simulink library "Library_ASK"  (R2018b)
settings: Solver=VariableStepAuto  StartTime=0.0  StopTime=10.0  RelTol=1e-3  EnableMultiTasking=on
undefined symbols (not defined in the file): akt_2GTR_az_HA, akt_2GTR_az_VA, akt_2GTR_rn_HA, akt_2GTR_rn_VA, akt_GTR_az_HA, akt_GTR_az_VA, akt_GTR_rn_HA, akt_GTR_rn_VA, alpha, b_zahn, beta_b, breakpointset, choose_ulg, DiscIntNeverNeededParam, eps_1, eps_2, eps_alpha, eta_aa, eta_Kegel_max, Fx_LSD_max, Fx_mUELG_max, i_DF, i_Kegelrad_OD, i_TRM_G1_HA, i_TRM_G1_VA, i_TRM_G2_HA, i_TRM_G2_VA, i_TRM_HA, i_TRM_Stufe_1_HA, i_TRM_Stufe_1_VA, i_TRM_Stufe_2_HA, i_TRM_Stufe_2_VA, i_TRM_VA, M_Cl_LSD_max, M_Cl_mUELG_max, M_EM_max, M_Kupplung_mUELG_Schlepp, mu_cl_LSD, mu_cl_mUELG, n_EM_max, n_Stufen_TRM_HA, n_Stufen_TRM_VA, ndyn_oil, nreib_LSD, nreib_mUELG, par_MDT, par_VEH, Ra, rm_LSD, rm_mUELG, select_Traktion_split, stepsize, wkg_Diff_mUELG, wkg_GTR, X_L, z_atts, z_ayc, z_ayc_lr, z_ayc_rl
libraries: simulink x23, $bdroot x6
(part 2 of 4)

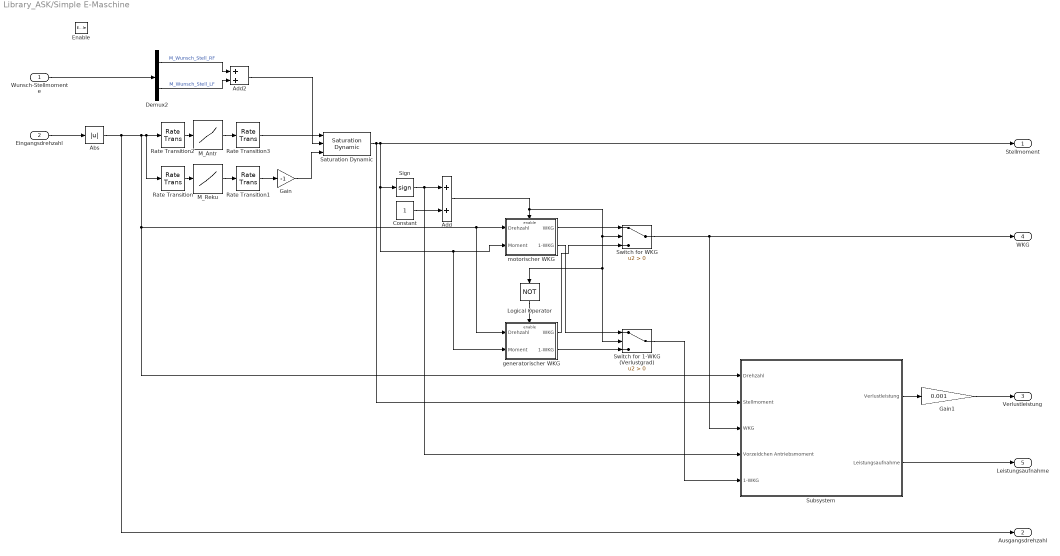
== system Library_ASK/Simple E-Maschine ==
  Wunsch-Stellmomente : Inport
  Eingangsdrehzahl : Inport  Port=2
  Enable : EnablePort
  Abs : Abs
  Add : Sum
  Add2 : Sum
  Constant : Constant
  Demux2 : Demux  Outputs=2
  Gain : Gain  Gain=-1
  Gain1 : Gain  Gain=0.001
  Logical Operator : Logic  Operator=NOT  AllPortsSameDT=off  OutDataTypeStr=boolean
  M_Antr : Lookup_n-D  NumberOfTableDimensions=1  BreakpointsForDimension1=Mot_nmax_Curve  Table=Mot_Mmax_Curve  ExtrapMethod=Clip  UseLastTableValue=on  InternalRulePriority=Speed  RndMeth=Simplest  InputSameDT=on
  M_Reku : Lookup_n-D  NumberOfTableDimensions=1  BreakpointsForDimension1=Gen_nmax_Curve  Table=Gen_Mmax_Curve  ExtrapMethod=Clip  UseLastTableValue=on  InternalRulePriority=Speed  RndMeth=Simplest  InputSameDT=on
  Rate Transition : RateTransition  OutPortSampleTime=stepsize*10
  Rate Transition1 : RateTransition  OutPortSampleTimeOpt=Inherit  OutPortSampleTime=0.001
  Rate Transition2 : RateTransition  OutPortSampleTime=stepsize*10
  Rate Transition3 : RateTransition  OutPortSampleTimeOpt=Inherit  OutPortSampleTime=0.001
  Saturation Dynamic : simulink/Discontinuities/Saturation Dynamic  OutMin=[]  OutMax=[]  OutDataTypeStr=Inherit: Same as second input  OutDataType=fixdt(1, 16)  OutScaling=2^-10  DoSatur=off
  Sign : Signum
  Subsystem : Subsystem
  Switch for 1-WKG (Verlustgrad) : Switch  Criteria=u2 > Threshold
  Switch for WKG : Switch  Criteria=u2 > Threshold
  generatorischer WKG : Subsystem
  motorischer WKG : Subsystem
  Stellmoment : Outport  InitialOutput=0
  Ausgangsdrehzahl : Outport  Port=2  InitialOutput=0
  Verlustleistung : Outport  Port=3
  WKG : Outport  Port=4
  Leistungsaufnahme : Outport  Port=5  InitialOutput=0
  wires:
  Switch for 1-WKG (Verlustgrad)/1 -> Subsystem/5(1-WKG)
  Subsystem/2(Leistungsaufnahme) -> Leistungsaufnahme/1
  Subsystem/1(Verlustleistung) -> Gain1/1
  Switch for WKG/1 -> WKG/1, Subsystem/3(WKG)
  Sign/1 -> Add/1, Subsystem/4(Vorzeidchen Antriebsmoment)
  Abs/1 -> Ausgangsdrehzahl/1, generatorischer WKG/1(Drehzahl), motorischer WKG/1(Drehzahl), Subsystem/1(Drehzahl), Rate Transition2/1, Rate Transition/1
  Logical Operator/1 -> generatorischer WKG/Enable
  Add/1 -> motorischer WKG/Enable, Switch for WKG/2, Logical Operator/1, Switch for 1-WKG (Verlustgrad)/2
  generatorischer WKG/2(1-WKG) -> Switch for 1-WKG (Verlustgrad)/3
  generatorischer WKG/1(WKG) -> Switch for WKG/3
  motorischer WKG/1(WKG) -> Switch for WKG/1
  Constant/1 -> Add/2
  motorischer WKG/2(1-WKG) -> Switch for 1-WKG (Verlustgrad)/1
  Gain/1 -> Saturation Dynamic/3
  Saturation Dynamic/1 -> Stellmoment/1, Sign/1, generatorischer WKG/2(Moment), motorischer WKG/2(Moment), Subsystem/2(Stellmoment)
  Eingangsdrehzahl/1 -> Abs/1
  Add2/1 -> Saturation Dynamic/2
  Demux2/2 -> Add2/2  "M_Wunsch_Stell_LF"
  Demux2/1 -> Add2/1  "M_Wunsch_Stell_RF"
  Wunsch-Stellmomente/1 -> Demux2/1
  Rate Transition3/1 -> Saturation Dynamic/1
  Rate Transition1/1 -> Gain/1
  Rate Transition2/1 -> M_Antr/1
  M_Antr/1 -> Rate Transition3/1
  Rate Transition/1 -> M_Reku/1
  M_Reku/1 -> Rate Transition1/1
  Gain1/1 -> Verlustleistung/1

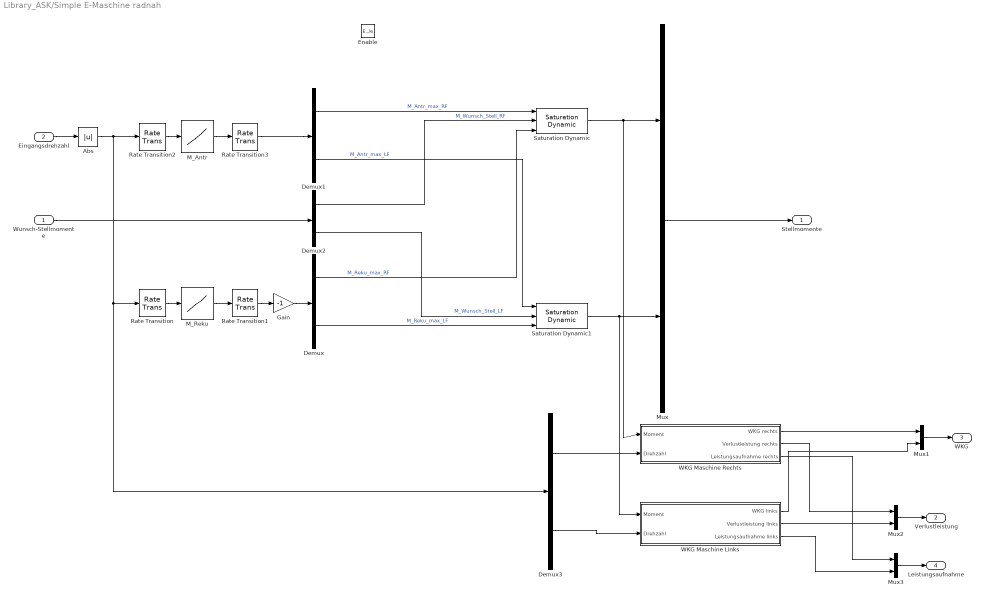
== system Library_ASK/Simple E-Maschine radnah ==
  Wunsch-Stellmomente : Inport
  Eingangsdrehzahl : Inport  Port=2
  Enable : EnablePort
  Abs : Abs
  Demux{,1..3} (4 alike) : Demux  Outputs=2
  Gain : Gain  Gain=-1
  M_Antr : Lookup_n-D  NumberOfTableDimensions=1  BreakpointsForDimension1=Mot_nmax_Curve  Table=Mot_Mmax_Curve  ExtrapMethod=Clip  UseLastTableValue=on  InternalRulePriority=Speed  RndMeth=Simplest  InputSameDT=on
  M_Reku : Lookup_n-D  NumberOfTableDimensions=1  BreakpointsForDimension1=Gen_nmax_Curve  Table=Gen_Mmax_Curve  ExtrapMethod=Clip  UseLastTableValue=on  InternalRulePriority=Speed  RndMeth=Simplest  InputSameDT=on
  Mux{,1..3} (4 alike) : Mux  Inputs=2
  Rate Transition : RateTransition  OutPortSampleTime=stepsize*10
  Rate Transition1 : RateTransition  OutPortSampleTimeOpt=Inherit  OutPortSampleTime=0.001
  Rate Transition2 : RateTransition  OutPortSampleTime=stepsize*10
  Rate Transition3 : RateTransition  OutPortSampleTimeOpt=Inherit  OutPortSampleTime=0.001
  Saturation Dynamic : simulink/Discontinuities/Saturation Dynamic  OutMin=[]  OutMax=[]  OutDataTypeStr=Inherit: Same as second input  OutDataType=fixdt(1, 16)  OutScaling=2^-10  DoSatur=off
  Saturation Dynamic1 : simulink/Discontinuities/Saturation Dynamic  OutMin=[]  OutMax=[]  OutDataTypeStr=Inherit: Same as second input  OutDataType=fixdt(1, 16)  OutScaling=2^-10  DoSatur=off
  WKG Maschine Links : Subsystem
  WKG Maschine Rechts : Subsystem
  Stellmomente : Outport  InitialOutput=0
  Verlustleistung : Outport  Port=2
  WKG : Outport  Port=3
  Leistungsaufnahme : Outport  Port=4
  wires:
  WKG Maschine Links/3(Leistungsaufnahme links) -> Mux3/2
  WKG Maschine Rechts/3(Leistungsaufnahme rechts) -> Mux3/1
  Mux3/1 -> Leistungsaufnahme/1
  Abs/1 -> Rate Transition2/1, Rate Transition/1, Demux3/1
  Mux2/1 -> Verlustleistung/1
  Demux3/2 -> WKG Maschine Links/2(Drehzahl)
  Demux3/1 -> WKG Maschine Rechts/2(Drehzahl)
  Mux1/1 -> WKG/1
  WKG Maschine Links/2(Verlustleistung links) -> Mux2/2
  WKG Maschine Rechts/2(Verlustleistung rechts) -> Mux2/1
  WKG Maschine Rechts/1(WKG rechts) -> Mux1/1
  WKG Maschine Links/1(WKG links) -> Mux1/2
  Gain/1 -> Demux/1
  Eingangsdrehzahl/1 -> Abs/1
  M_Reku/1 -> Rate Transition1/1
  Rate Transition/1 -> M_Reku/1
  M_Antr/1 -> Rate Transition3/1
  Rate Transition2/1 -> M_Antr/1
  Rate Transition1/1 -> Gain/1
  Rate Transition3/1 -> Demux1/1
  Demux/1 -> Saturation Dynamic/3  "M_Reku_max_RF"
  Demux/2 -> Saturation Dynamic1/3  "M_Reku_max_LF"
  Demux1/1 -> Saturation Dynamic/1  "M_Antr_max_RF"
  Demux1/2 -> Saturation Dynamic1/1  "M_Antr_max_LF"
  Wunsch-Stellmomente/1 -> Demux2/1
  Demux2/1 -> Saturation Dynamic/2  "M_Wunsch_Stell_RF"
  Demux2/2 -> Saturation Dynamic1/2  "M_Wunsch_Stell_LF"
  Saturation Dynamic/1 -> Mux/1, WKG Maschine Rechts/1(Moment)
  Saturation Dynamic1/1 -> Mux/2, WKG Maschine Links/1(Moment)
  Mux/1 -> Stellmomente/1

== system Library_ASK/Simple E-Maschine radnah ALT ==
  Wunsch-Stellmomente : Inport
  Eingangsdrehzahl : Inport  Port=2
  Enable : EnablePort
  Abs : Abs
  Demux{,1..3} (4 alike) : Demux  Outputs=2
  Gain : Gain  Gain=-1
  M_Antr : Lookup_n-D  NumberOfTableDimensions=1  BreakpointsForDimension1=Mot_nmax_Curve  Table=Mot_Mmax_Curve  ExtrapMethod=Clip  UseLastTableValue=on  InternalRulePriority=Speed  RndMeth=Simplest  InputSameDT=on
  M_Reku : Lookup_n-D  NumberOfTableDimensions=1  BreakpointsForDimension1=Gen_nmax_Curve  Table=Gen_Mmax_Curve  ExtrapMethod=Clip  UseLastTableValue=on  InternalRulePriority=Speed  RndMeth=Simplest  InputSameDT=on
  Mux{,1..3} (4 alike) : Mux  Inputs=2
  Rate Transition : RateTransition  OutPortSampleTime=stepsize*10
  Rate Transition1 : RateTransition  OutPortSampleTimeOpt=Inherit  OutPortSampleTime=0.001
  Rate Transition2 : RateTransition  OutPortSampleTime=stepsize*10
  Rate Transition3 : RateTransition  OutPortSampleTimeOpt=Inherit  OutPortSampleTime=0.001
  Saturation Dynamic : simulink/Discontinuities/Saturation Dynamic  OutMin=[]  OutMax=[]  OutDataTypeStr=Inherit: Same as second input  OutDataType=fixdt(1, 16)  OutScaling=2^-10  DoSatur=off
  Saturation Dynamic1 : simulink/Discontinuities/Saturation Dynamic  OutMin=[]  OutMax=[]  OutDataTypeStr=Inherit: Same as second input  OutDataType=fixdt(1, 16)  OutScaling=2^-10  DoSatur=off
  WKG Maschine Links : Subsystem
  WKG Maschine Rechts : Subsystem
  Stellmomente : Outport  InitialOutput=0
  Verlustleistung : Outport  Port=2
  WKG : Outport  Port=3
  Leistungsaufnahme : Outport  Port=4
  wires:
  Mux/1 -> Stellmomente/1
  Saturation Dynamic1/1 -> WKG Maschine Links/1(Moment), Mux/2
  Saturation Dynamic/1 -> WKG Maschine Rechts/1(Moment), Mux/1
  Demux2/2 -> Saturation Dynamic1/2  "M_Wunsch_Stell_LF"
  Demux2/1 -> Saturation Dynamic/2  "M_Wunsch_Stell_RF"
  Wunsch-Stellmomente/1 -> Demux2/1
  Demux1/2 -> Saturation Dynamic1/1  "M_Antr_max_LF"
  Demux1/1 -> Saturation Dynamic/1  "M_Antr_max_RF"
  Demux/2 -> Saturation Dynamic1/3  "M_Reku_max_LF"
  Demux/1 -> Saturation Dynamic/3  "M_Reku_max_RF"
  Rate Transition3/1 -> Demux1/1
  Rate Transition1/1 -> Gain/1
  Rate Transition2/1 -> M_Antr/1
  M_Antr/1 -> Rate Transition3/1
  Rate Transition/1 -> M_Reku/1
  M_Reku/1 -> Rate Transition1/1
  Eingangsdrehzahl/1 -> Abs/1
  Gain/1 -> Demux/1
  WKG Maschine Links/1(WKG links) -> Mux1/2
  WKG Maschine Rechts/1(WKG rechts) -> Mux1/1
  WKG Maschine Rechts/2(Verlustleistung rechts) -> Mux2/1
  WKG Maschine Links/2(Verlustleistung links) -> Mux2/2
  Mux1/1 -> WKG/1
  Demux3/1 -> WKG Maschine Rechts/2(Drehzahl)
  Demux3/2 -> WKG Maschine Links/2(Drehzahl)
  Mux2/1 -> Verlustleistung/1
  Abs/1 -> Demux3/1, Rate Transition/1, Rate Transition2/1
  Mux3/1 -> Leistungsaufnahme/1
  WKG Maschine Rechts/3(Leistungsaufnahme rechts) -> Mux3/1
  WKG Maschine Links/3(Leistungsaufnahme links) -> Mux3/2

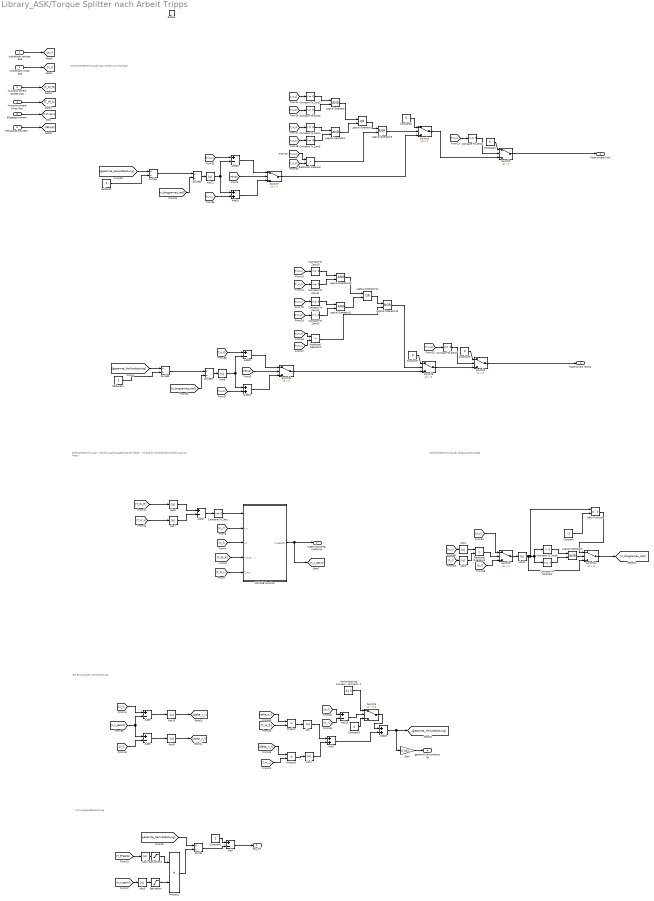
== system Library_ASK/Torque Splitter nach Arbeit Tripps ==
  note: Drehzahlberechnung des langsameren Rades
  note: Drehzahlbestimmung - welche Kupplung geschlossen bleibt - wichtig für die Drehzahlrückführung zum Motor
  note: Berechnung der Verlustleistung
  note: Wirkungsgradberechnung
  note: Momentenberechnung für das rechte und linke Rad
  Istdrehzahl rechtes Rad : Inport
  Istdrehzahl linkes Rad : Inport  Port=2
  Wunschmoment rechtes Rad : Inport  Port=3
  Wunschmoment linkes Rad : Inport  Port=4
  Eingangsmoment : Inport  Port=5
  Rekuperationsindex : Inport  Port=6
  Enable : EnablePort
  Abs{,1..12} (13 alike) : Abs
  Add{,8..9,13,16..17,20} (7 alike) : Sum  Inputs=+-
  Add{7,18..19,21} (4 alike) : Sum
  Compare To Constant : simulink/Logic and Bit Operations/Compare To Constant  relop=<=  const=1  OutDataTypeStr=boolean
  Compare To Zero : simulink/Logic and Bit Operations/Compare To Zero  relop=~=  OutDataTypeStr=boolean
  Compare To Zero1 : simulink/Logic and Bit Operations/Compare To Zero  relop===  OutDataTypeStr=boolean
  Compare To Zero{2..3,10..11} (4 alike) : simulink/Logic and Bit Operations/Compare To Zero  relop=<=  OutDataTypeStr=boolean
  Compare To Zero{4..5,12..13} (4 alike) : simulink/Logic and Bit Operations/Compare To Zero  relop=>=  OutDataTypeStr=boolean
  Compare To Zero7 : simulink/Logic and Bit Operations/Compare To Zero  relop===  OutDataTypeStr=boolean
  Compare To Zero9 : simulink/Logic and Bit Operations/Compare To Zero  relop=>  OutDataTypeStr=boolean
  Constant : Constant  Value=-1
  Constant1 : Constant
  Constant{2,4,6..7,9} (5 alike) : Constant  Value=0
  Divide{,1..3,5} (5 alike) : Product  Inputs=*/
  Gain : Gain  Gain=0.001
  Logical Operator{,1,3,10..11} (5 alike) : Logic  AllPortsSameDT=off  OutDataTypeStr=boolean
  Logical Operator12 : Logic  Operator=OR  AllPortsSameDT=off  OutDataTypeStr=boolean
  Logical Operator13 : Logic  Operator=NOR  AllPortsSameDT=off  OutDataTypeStr=boolean
  Logical Operator2 : Logic  Operator=OR  AllPortsSameDT=off  OutDataTypeStr=boolean
  Logical Operator5 : Logic  Operator=NOR  AllPortsSameDT=off  OutDataTypeStr=boolean
  MATLAB Function : MATLAB Function  TreatAsAtomicUnit=on
  Math Function : Math  Operator=pow  SaturateOnIntegerOverflow=on
  Product : Product
  Product1 : Product
  Product2 : Product
  Relational Operator : RelationalOperator  Operator=>  OutDataTypeStr=boolean  RndMeth=Simplest
  Relational Operator2 : RelationalOperator  Operator=>  OutDataTypeStr=boolean  RndMeth=Simplest
  Relational Operator3 : RelationalOperator  Operator=<  OutDataTypeStr=boolean  RndMeth=Simplest
  Saturation : Saturate  UpperLimit=100000000000  LowerLimit=0.01
  Saturation1 : Saturate  UpperLimit=100000000000  LowerLimit=0.01
  Switch{1..3,6..9,11} (8 alike) : Switch  Criteria=u2 > Threshold
  Switch5 : Switch  Criteria=u2 ~= 0
  "Verlustleistung Aktuierung muss immer aufgebracht werden [W], nur bei Fahrt aktiv 1" : Constant  Value=41.3
  halbieren : Constant  Value=2
  halbieren1 : Constant  Value=2
  Radmoment rechts : Outport
  "Radmoment links " : Outport  Port=2
  n_geschlossene_Kupplung : Outport  Port=3
  gesamte Verlustleistung : Outport  Port=4
  eta_TS : Outport  Port=5
  wires:
  Istdrehzahl linkes Rad/1 -> [n_l]
  Istdrehzahl rechtes Rad/1 -> [n_r]
  Eingangsmoment/1 -> [T_Eingang]
  Wunschmoment rechtes Rad/1 -> [T_W_R]
  Wunschmoment linkes Rad/1 -> [T_W_L]
  [n_l] -> Switch3/3
  [n_r] -> Switch3/1
  Relational Operator3/1 -> Switch3/2
  Switch5/1 -> Add18/1
  [gesamte_Verlustleistung] -> Divide/1
  [delta_n_r] -> Product/1
  [n_k_geschl] -> Add8/1, Add9/2
  [T_Eingang] -> Abs1/1
  [T_W_R] -> Product/2
  [n_l] -> Add8/2
  Abs9/1 -> [delta_n_l]
  "Verlustleistung Aktuierung muss immer aufgebracht werden [W], nur bei Fahrt aktiv 1"/1 -> Switch5/1
  Add/1 -> eta_TS/1
  Product/1 -> Abs/1
  [n_r] -> Add13/2
  [T_W_L] -> Product1/2
  Abs2/1 -> Add7/2
  [n_l] -> Add13/1
  Product1/1 -> Abs2/1
  Abs10/1 -> [delta_n_r]
  [n_r] -> Add9/1
  Constant9/1 -> Switch5/3
  Add18/1 -> Gain/1, [gesamte_Verlustleistung]
  Add7/1 -> Add18/2
  Add9/1 -> Abs10/1
  Constant1/1 -> Add/1
  [delta_n_l] -> Product1/1
  [n_k_geschl] -> Abs3/1
  Product2/1 -> Divide/2
  Add8/1 -> Abs9/1
  Abs/1 -> Add7/1
  Divide/1 -> Add/2
  Add13/1 -> Switch5/2
  [n_langsames_rad] -> Divide3/2
  [T_W_R] -> Add20/1
  [T_W_L] -> Add19/2
  Divide3/1 -> Abs8/1
  Add19/1 -> Switch7/3
  Divide2/1 -> Abs11/1
  halbieren1/1 -> Divide5/2
  [gesamte_Verlustleistung] -> Divide5/1
  Divide5/1 -> Divide3/1
  [T_W_R] -> Add21/2
  Add20/1 -> Switch6/1
  Add16/1 -> Switch7/1
  halbieren/1 -> Divide1/2
  [T_W_L] -> Add16/1
  Add21/1 -> Switch6/3
  [rekup] -> Switch6/2
  [n_langsames_rad] -> Divide2/2
  [rekup] -> Switch7/2
  [gesamte_Verlustleistung] -> Divide1/1
  Divide1/1 -> Divide2/1
  Rekuperationsindex/1 -> [rekup]
  [T_W_L] -> Abs7/1
  Compare To Zero/1 -> MATLAB Function/1(u)
  Add17/1 -> Compare To Zero/1
  MATLAB Function/1(n_k_geschl) -> [n_k_geschl], n_geschlossene_Kupplung/1
  [T_W_R] -> Abs6/1
  Abs6/1 -> Add17/1
  Abs7/1 -> Add17/2
  Gain/1 -> gesamte Verlustleistung/1
  Switch2/1 -> "Radmoment links "/1
  [T_W_R] -> Compare To Zero3/1
  [T_W_R] -> Relational Operator/2
  [T_W_L] -> Compare To Zero2/1
  Logical Operator2/1 -> Logical Operator5/1
  Compare To Zero5/1 -> Logical Operator1/2
  Logical Operator1/1 -> Logical Operator2/2
  [T_W_L] -> Relational Operator/1
  Relational Operator/1 -> Logical Operator5/2
  Compare To Zero3/1 -> Logical Operator/2
  Logical Operator/1 -> Logical Operator2/1
  Constant2/1 -> Switch1/1
  Compare To Zero2/1 -> Logical Operator/1
  [T_W_L] -> Compare To Zero4/1
  Logical Operator5/1 -> Switch1/2
  Switch7/1 -> Switch1/3
  Switch1/1 -> Switch2/3
  Compare To Zero1/1 -> Switch2/2
  [T_W_L] -> Compare To Zero1/1
  [T_W_R] -> Compare To Zero5/1
  Compare To Zero4/1 -> Logical Operator1/1
  Constant4/1 -> Switch2/1
  Switch9/1 -> Radmoment rechts/1
  Compare To Zero7/1 -> Switch9/2
  Constant6/1 -> Switch9/1
  Switch6/1 -> Switch8/3
  Switch8/1 -> Switch9/3
  Logical Operator11/1 -> Logical Operator12/2
  [T_W_L] -> Compare To Zero10/1
  [T_W_R] -> Compare To Zero11/1
  [T_W_R] -> Compare To Zero7/1
  Compare To Zero11/1 -> Logical Operator10/2
  Relational Operator2/1 -> Logical Operator13/2
  Logical Operator12/1 -> Logical Operator13/1
  [T_W_L] -> Compare To Zero12/1
  Logical Operator13/1 -> Switch8/2
  [T_W_R] -> Relational Operator2/1
  Compare To Zero13/1 -> Logical Operator11/2
  Compare To Zero10/1 -> Logical Operator10/1
  Logical Operator10/1 -> Logical Operator12/1
  [T_W_L] -> Relational Operator2/2
  [T_W_R] -> Compare To Zero13/1
  Constant7/1 -> Switch8/1
  Compare To Zero12/1 -> Logical Operator11/1
  Abs3/1 -> Saturation/1
  Saturation/1 -> Product2/2
  Abs1/1 -> Saturation1/1
  Saturation1/1 -> Product2/1
  [n_r] -> Abs4/1
  Abs4/1 -> Relational Operator3/1
  [n_l] -> Abs5/1
  Abs5/1 -> Relational Operator3/2
  [T_W_L] -> MATLAB Function/5(T_W_L)
  [T_W_R] -> MATLAB Function/4(T_W_R)
  [n_l] -> MATLAB Function/3(n_l)
  [n_r] -> MATLAB Function/2(n_r)
  Abs8/1 -> Add21/1, Add20/2
  Abs11/1 -> Add16/2, Add19/1
  Switch3/1 -> Abs12/1
  Compare To Zero9/1 -> Logical Operator3/1
  Compare To Constant/1 -> Logical Operator3/2
  Logical Operator3/1 -> Switch11/2
  Math Function/1 -> Switch11/1
  Constant/1 -> Math Function/2
  Abs12/1 -> Switch11/3, Math Function/1, Compare To Zero9/1, Compare To Constant/1
  Switch11/1 -> [n_langsames_rad]

== system Library_ASK/Torque Splitter v2 C. Angerer 10//2018 ==
  Istdrehzahl rechtes Rad : Inport
  Istdrehzahl linkes Rad : Inport  Port=2
  Wunschmoment rechtes Rad : Inport  Port=3
  Wunschmoment linkes Rad : Inport  Port=4
  Eingangsmoment : Inport  Port=5
  Rekuindex : Inport  Port=6
  Enable : EnablePort
  Constant : Constant  Value=select_Traktion_split
  Gain : Gain  Gain=0.001
  MATLAB Function : MATLAB Function  TreatAsAtomicUnit=on
  MATLAB Function2 : MATLAB Function  TreatAsAtomicUnit=on
  Terminator : Terminator
  Radmoment rechts : Outport
  "Radmoment links " : Outport  Port=2
  n_geschlossene_Kupplung : Outport  Port=3
  gesamte Verlustleistung : Outport  Port=4
  eta_TS : Outport  Port=5
  wires:
  MATLAB Function/3(P_loss_TS) -> Gain/1
  Rekuindex/1 -> Terminator/1
  MATLAB Function/1(M_rad_r) -> Radmoment rechts/1
  MATLAB Function/2(M_rad_l) -> "Radmoment links "/1
  Gain/1 -> gesamte Verlustleistung/1
  MATLAB Function/4(eta_TS) -> eta_TS/1
  MATLAB Function2/1(n_k_geschl) -> n_geschlossene_Kupplung/1, MATLAB Function/6(n_k_geschl)
  Istdrehzahl rechtes Rad/1 -> MATLAB Function2/1(n_r), MATLAB Function/1(n_r)
  Istdrehzahl linkes Rad/1 -> MATLAB Function2/2(n_l), MATLAB Function/2(n_l)
  Wunschmoment rechtes Rad/1 -> MATLAB Function/3(T_W_R)
  Wunschmoment linkes Rad/1 -> MATLAB Function/4(T_W_L)
  Eingangsmoment/1 -> MATLAB Function/5(M_Getriebeausgang), MATLAB Function2/3(Eingangsmoment)
  Constant/1 -> MATLAB Function2/4(split)

== system Library_ASK/Zweigängiges Getriebe az HA ==
  note: Lastanteil
  Eingangsmoment : Inport
  Eingangsdrehzahl : Inport  Port=2
  Enable : EnablePort
  Abs3 : Abs
  Constant : Constant  Value=n_Stufen_TRM_HA
  Constant1 : Constant  Value=M_EM_max
  Constant2 : Constant  Value=i_TRM_G2_HA
  Constant3 : Constant  Value=i_TRM_G1_HA
  Constant5 : Constant  Value=n_EM_max
  Divide : Product  Inputs=*/
  Lastanteil : Product  Inputs=*/
  MATLAB Function : MATLAB Function  TreatAsAtomicUnit=on
  Product : Product  Inputs=3
  Product4 : Product
  Subsystem : Subsystem
  Terminator : Terminator
  WKG : Subsystem
  Ausgangsmoment : Outport  InitialOutput=0
  Energieverlust : Outport  Port=2  InitialOutput=0
  Verlustleistung : Outport  Port=3
  eta_GTR : Outport  Port=4
  wires:
  Constant/1 -> WKG/2(Stufenanzahl)
  MATLAB Function/1(i_TRM) -> WKG/1(Stufenübersetzung), Divide/2, Product/2
  Constant5/1 -> MATLAB Function/2(n_EM_max)
  Constant3/1 -> MATLAB Function/3(i_TRM_G1)
  Constant2/1 -> MATLAB Function/4(i_TRM_G2)
  Eingangsdrehzahl/1 -> MATLAB Function/1(n_EM), Product4/2, Divide/1, WKG/3(Eingangsdrehzahl)
  Subsystem/2(Verlustleistung [kW]) -> Verlustleistung/1
  Subsystem/1(Energieverlust [kWh]) -> Energieverlust/1
  Product4/1 -> Subsystem/2(Inputleistung)  "Electric Motor Input Power [W]"
  Abs3/1 -> WKG/4(Last)
  Constant1/1 -> Lastanteil/2
  Lastanteil/1 -> Abs3/1
  Product/1 -> Ausgangsmoment/1
  Eingangsmoment/1 -> Lastanteil/1, Product/1, Product4/1
  WKG/1(WKG) -> eta_GTR/1, Product/3, Subsystem/1(WKG)
  Divide/1 -> Terminator/1

== system Library_ASK/Zweigängiges Getriebe az VA ==
  note: Lastanteil
  Eingangsmoment : Inport
  Eingangsdrehzahl : Inport  Port=2
  Enable : EnablePort
  Abs3 : Abs
  Constant : Constant  Value=n_Stufen_TRM_VA
  Constant1 : Constant  Value=M_EM_max
  Constant3 : Constant  Value=i_TRM_G1_VA
  Divide : Product  Inputs=*/
  Lastanteil : Product  Inputs=*/
  Product : Product  Inputs=3
  Product4 : Product
  Subsystem : Subsystem
  Terminator : Terminator
  WKG : Subsystem
  Ausgangsmoment : Outport  InitialOutput=0
  Energieverlust : Outport  Port=2  InitialOutput=0
  Verlustleistung : Outport  Port=3
  eta_GTR : Outport  Port=4
  wires:
  Divide/1 -> Terminator/1
  WKG/1(WKG) -> Subsystem/1(WKG), Product/3, eta_GTR/1
  Eingangsmoment/1 -> Product4/1, Product/1, Lastanteil/1
  Product/1 -> Ausgangsmoment/1
  Lastanteil/1 -> Abs3/1
  Constant1/1 -> Lastanteil/2
  Abs3/1 -> WKG/4(Last)
  Product4/1 -> Subsystem/2(Inputleistung)  "Electric Motor Input Power [W]"
  Subsystem/1(Energieverlust [kWh]) -> Energieverlust/1
  Subsystem/2(Verlustleistung [kW]) -> Verlustleistung/1
  Eingangsdrehzahl/1 -> WKG/3(Eingangsdrehzahl), Divide/1, Product4/2
  ? -> ?
  Constant3/1 -> ?
  ? -> Product/2, Divide/2, WKG/1(Stufenübersetzung)
  Constant/1 -> WKG/2(Stufenanzahl)

== system Library_ASK/Zweigängiges Getriebe rn HA ==
  note: Lastanteil
  Eingangsmoment : Inport
  Eingangsdrehzahl : Inport  Port=2
  Enable : EnablePort
  Abs3 : Abs
  Constant : Constant  Value=n_Stufen_TRM_HA
  Constant1 : Constant  Value=M_EM_max
  Constant2 : Constant  Value=i_TRM_G2_HA
  Constant3 : Constant  Value=i_TRM_G1_HA
  Constant5 : Constant  Value=n_EM_max
  Demux : Demux  Outputs=2
  Divide : Product  Inputs=*/
  Lastanteil : Product  Inputs=*/
  MATLAB Function : MATLAB Function  TreatAsAtomicUnit=on
  MATLAB Function1 : MATLAB Function  TreatAsAtomicUnit=on
  Mux : Mux  Inputs=2
  Product : Product  Inputs=3
  Product4 : Product
  Subsystem : Subsystem
  Terminator : Terminator
  WKG : Subsystem
  Ausgangsmoment : Outport  InitialOutput=0
  Energieverlust : Outport  Port=2  InitialOutput=0
  Verlustleistung : Outport  Port=3
  eta_GTR : Outport  Port=4
  wires:
  Mux/1 -> Product/2, Divide/2, WKG/1(Stufenübersetzung)
  MATLAB Function1/1(i_TRM) -> Mux/2
  MATLAB Function/1(i_TRM) -> Mux/1
  Demux/2 -> MATLAB Function1/1(n_EM)
  Demux/1 -> MATLAB Function/1(n_EM)
  Eingangsdrehzahl/1 -> Demux/1, Product4/2, Divide/1, WKG/3(Eingangsdrehzahl)
  Divide/1 -> Terminator/1
  WKG/1(WKG) -> Subsystem/1(WKG), Product/3, eta_GTR/1
  Eingangsmoment/1 -> Lastanteil/1, Product4/1, Product/1
  Product/1 -> Ausgangsmoment/1
  Lastanteil/1 -> Abs3/1
  Constant1/1 -> Lastanteil/2
  Abs3/1 -> WKG/4(Last)
  Product4/1 -> Subsystem/2(Inputleistung)  "Electric Motor Input Power [W]"
  Subsystem/1(Energieverlust [kWh]) -> Energieverlust/1
  Subsystem/2(Verlustleistung [kW]) -> Verlustleistung/1
  Constant2/1 -> MATLAB Function/4(i_TRM_G2), MATLAB Function1/4(i_TRM_G2)
  Constant3/1 -> MATLAB Function/3(i_TRM_G1), MATLAB Function1/3(i_TRM_G1)
  Constant5/1 -> MATLAB Function/2(n_EM_max), MATLAB Function1/2(n_EM_max)
  Constant/1 -> WKG/2(Stufenanzahl)

== system Library_ASK/Zweigängiges Getriebe rn VA ==
  note: Lastanteil
  Eingangsmoment : Inport
  Eingangsdrehzahl : Inport  Port=2
  Enable : EnablePort
  Abs3 : Abs
  Constant : Constant  Value=n_Stufen_TRM_VA
  Constant1 : Constant  Value=M_EM_max
  Constant2 : Constant  Value=i_TRM_G2_VA
  Constant3 : Constant  Value=i_TRM_G1_VA
  Constant5 : Constant  Value=n_EM_max
  Demux : Demux  Outputs=2
  Divide : Product  Inputs=*/
  Lastanteil : Product  Inputs=*/
  MATLAB Function : MATLAB Function  TreatAsAtomicUnit=on
  MATLAB Function1 : MATLAB Function  TreatAsAtomicUnit=on
  Mux : Mux  Inputs=2
  Product : Product  Inputs=3
  Product4 : Product
  Subsystem : Subsystem
  Terminator : Terminator
  WKG : Subsystem
  Ausgangsmoment : Outport  InitialOutput=0
  Energieverlust : Outport  Port=2  InitialOutput=0
  Verlustleistung : Outport  Port=3
  eta_GTR : Outport  Port=4
  wires:
  Constant/1 -> WKG/2(Stufenanzahl)
  Constant5/1 -> MATLAB Function1/2(n_EM_max), MATLAB Function/2(n_EM_max)
  Constant3/1 -> MATLAB Function1/3(i_TRM_G1), MATLAB Function/3(i_TRM_G1)
  Constant2/1 -> MATLAB Function1/4(i_TRM_G2), MATLAB Function/4(i_TRM_G2)
  Subsystem/2(Verlustleistung [kW]) -> Verlustleistung/1
  Subsystem/1(Energieverlust [kWh]) -> Energieverlust/1
  Product4/1 -> Subsystem/2(Inputleistung)  "Electric Motor Input Power [W]"
  Abs3/1 -> WKG/4(Last)
  Constant1/1 -> Lastanteil/2
  Lastanteil/1 -> Abs3/1
  Product/1 -> Ausgangsmoment/1
  Eingangsmoment/1 -> Product/1, Product4/1, Lastanteil/1
  WKG/1(WKG) -> eta_GTR/1, Product/3, Subsystem/1(WKG)
  Divide/1 -> Terminator/1
  Eingangsdrehzahl/1 -> WKG/3(Eingangsdrehzahl), Divide/1, Product4/2, Demux/1
  Demux/1 -> MATLAB Function/1(n_EM)
  Demux/2 -> MATLAB Function1/1(n_EM)
  MATLAB Function/1(i_TRM) -> Mux/1
  MATLAB Function1/1(i_TRM) -> Mux/2
  Mux/1 -> WKG/1(Stufenübersetzung), Divide/2, Product/2

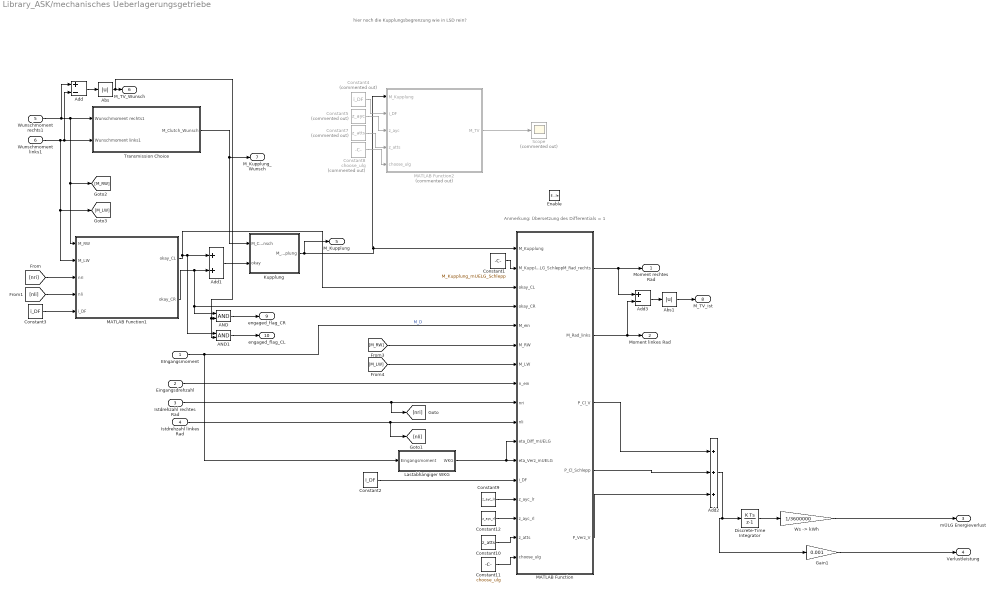
== system Library_ASK/mechanisches Ueberlagerungsgetriebe ==
  note: hier noch die Kupplungsbegrenzung wie in LSD rein?
  note: Anmerkung: Übersetzung des Differentials = 1
  EIngangsmoment : Inport
  Eingangsdrehzahl : Inport  Port=2
  Istdrehzahl rechtes Rad : Inport  Port=3
  Istdrehzahl linkes Rad : Inport  Port=4
  Wunschmoment rechts1 : Inport  Port=5
  Wunschmoment links1 : Inport  Port=6
  Enable : EnablePort
  AND : Logic  IconShape=distinctive  AllPortsSameDT=off  OutDataTypeStr=boolean
  AND1 : Logic  IconShape=distinctive  AllPortsSameDT=off  OutDataTypeStr=boolean
  Abs : Abs
  Abs1 : Abs
  Add : Sum  Inputs=+-
  Add1 : Sum
  Add2 : Sum  Inputs=+++
  Add3 : Sum  Inputs=+-
  Constant1 : Constant  Value=M_Kupplung_mUELG_Schlepp
  Constant10 : Constant  Value=z_atts
  Constant11 : Constant  Value=choose_ulg
  Constant12 : Constant  Value=z_ayc_rl
  Constant2 : Constant  Value=i_DF
  Constant3 : Constant  Value=i_DF
  Constant4 : Constant  Commented=on  Value=i_DF
  Constant5 : Constant  Commented=on  Value=z_ayc
  Constant7 : Constant  Commented=on  Value=z_atts
  Constant8 : Constant  Commented=on  Value=choose_ulg
  Constant9 : Constant  Value=z_ayc_lr
  Discrete-Time Integrator : DiscreteIntegrator  gainval=1  SampleTime=-1  ICPrevOutput=DiscIntNeverNeededParam  ICPrevScaledInput=DiscIntNeverNeededParam
  Gain1 : Gain  Gain=0.001
  Kupplung : Subsystem
  Lastabhängiger WKG : Subsystem
  MATLAB Function : MATLAB Function  TreatAsAtomicUnit=on
  MATLAB Function1 : MATLAB Function  TreatAsAtomicUnit=on
  MATLAB Function2 : MATLAB Function  Commented=on  TreatAsAtomicUnit=on
  Scope : Scope  Commented=on
  Transmission Choice : Subsystem
  "Ws -> kWh" : Gain  Gain=1/3600000
  Moment rechtes Rad : Outport  InitialOutput=0
  Moment linkes Rad : Outport  Port=2  InitialOutput=0
  mÜLG Energieverlust : Outport  Port=3  InitialOutput=0
  Verlustleistung : Outport  Port=4
  M_Kupplung : Outport  Port=5
  M_TV_Wunsch : Outport  Port=6
  M_Kupplung_Wunsch : Outport  Port=7
  M_TV_ist : Outport  Port=8
  engaged_flag_CR : Outport  Port=9
  engaged_flag_CL : Outport  Port=10
  wires:
  MATLAB Function/2(M_Rad_links) -> Add3/2, Moment linkes Rad/1
  MATLAB Function/1(M_Rad_rechts) -> Add3/1, Moment rechtes Rad/1
  Istdrehzahl rechtes Rad/1 -> [nri], MATLAB Function/9(nri)
  Istdrehzahl linkes Rad/1 -> [nli], MATLAB Function/10(nli)
  Constant2/1 -> MATLAB Function/13(i_DF)
  Discrete-Time Integrator/1 -> "Ws -> kWh"/1
  "Ws -> kWh"/1 -> mÜLG Energieverlust/1
  MATLAB Function/3(P_Cl_V) -> Add2/1
  EIngangsmoment/1 -> Lastabhängiger WKG/1(Eingangsmoment), MATLAB Function/5(M_ein)  "M_D"
  Eingangsdrehzahl/1 -> MATLAB Function/8(n_ein)
  Gain1/1 -> Verlustleistung/1
  MATLAB Function1/2(okay_CR) -> Add1/2, AND/1, MATLAB Function/4(okay_CR)
  MATLAB Function1/1(okay_CL) -> MATLAB Function/3(okay_CL), AND1/1, Add1/1
  Add1/1 -> Kupplung/2(okay)
  Kupplung/1(M_Kupplung) -> MATLAB Function2/1(M_Kupplung), MATLAB Function/1(M_Kupplung), M_Kupplung/1
  MATLAB Function/4(P_Cl_Schlepp) -> Add2/2
  MATLAB Function/5(P_Verz_V) -> Add2/3
  Add2/1 -> Gain1/1, Discrete-Time Integrator/1
  [nri] -> MATLAB Function1/3(nri)
  [nli] -> MATLAB Function1/4(nli)
  Constant3/1 -> MATLAB Function1/5(i_DF)
  [M_RW] -> MATLAB Function/6(M_RW)
  [M_LW] -> MATLAB Function/7(M_LW)
  Constant1/1 -> MATLAB Function/2(M_Kupplung_mUELG_Schlepp)
  Wunschmoment rechts1/1 -> Add/1, MATLAB Function1/1(M_RW), [M_RW], Transmission Choice/1(Wunschmoment rechts1)
  Wunschmoment links1/1 -> [M_LW], MATLAB Function1/2(M_LW), Add/2, Transmission Choice/2(Wunschmoment links1)
  Transmission Choice/1(M_Clutch_Wunsch) -> M_Kupplung_Wunsch/1, Kupplung/1(M_Cl_Wunsch)
  Constant4/1 -> MATLAB Function2/2(i_DF)
  Constant5/1 -> MATLAB Function2/3(z_ayc)
  Constant7/1 -> MATLAB Function2/4(z_atts)
  Constant8/1 -> MATLAB Function2/5(choose_ulg)
  Constant9/1 -> MATLAB Function/14(z_ayc_lr)
  Constant10/1 -> MATLAB Function/16(z_atts)
  Constant11/1 -> MATLAB Function/17(choose_ulg)
  MATLAB Function2/1(M_TV) -> Scope/1
  Constant12/1 -> MATLAB Function/15(z_ayc_rl)
  Lastabhängiger WKG/1(WKG) -> MATLAB Function/11(eta_Diff_mUELG), MATLAB Function/12(eta_Verz_mUELG)
  Add/1 -> Abs/1
  Abs/1 -> AND1/2, AND/2, M_TV_Wunsch/1
  Add3/1 -> Abs1/1
  Abs1/1 -> M_TV_ist/1
  AND1/1 -> engaged_flag_CL/1
  AND/1 -> engaged_flag_CR/1

== system Library_ASK/Drehzahlrückführung az HA/Fall Einganggetriebe ==
  Mittlere Raddrehzahl : Inport
  Enable : EnablePort
  Constant : Constant  Value=i_TRM_HA
  Divide : Product  Inputs=**
  Motordrehzahl : Outport
  wires:
  Divide/1 -> Motordrehzahl/1
  Mittlere Raddrehzahl/1 -> Divide/1
  Constant/1 -> Divide/2

== system Library_ASK/Drehzahlrückführung az HA/Fall Zweiganggetriebe ==
  note: auf diese Weise wird die Goto/From - Rückführung aus dem EM -Block überflüssig
  Mittlere Raddrehzahl : Inport
  Enable : EnablePort
  Constant : Constant  Value=i_TRM_G1_HA
  Constant1 : Constant  Value=i_TRM_G2_HA
  Constant2 : Constant  Value=n_EM_max
  Divide : Product  Inputs=**
  Divide1 : Product  Inputs=**
  MATLAB Function : MATLAB Function  TreatAsAtomicUnit=on
  Motordrehzahl : Outport
  wires:
  Constant/1 -> MATLAB Function/3(i_TRM_G1), Divide/2
  Mittlere Raddrehzahl/1 -> Divide/1, Divide1/1
  MATLAB Function/1(i_TRM) -> Divide1/2
  Divide/1 -> MATLAB Function/1(n_EM)  "Motordrehzahl wenn im ersten Gang"
  Constant1/1 -> MATLAB Function/4(i_TRM_G2)
  Divide1/1 -> Motordrehzahl/1
  Constant2/1 -> MATLAB Function/2(n_EM_max)

== system Library_ASK/Drehzahlrückführung az VA/Fall Einganggetriebe ==
  Mittlere Raddrehzahl : Inport
  Enable : EnablePort
  Constant : Constant  Value=i_TRM_VA
  Divide : Product  Inputs=**
  Motordrehzahl : Outport
  wires:
  Constant/1 -> Divide/2
  Mittlere Raddrehzahl/1 -> Divide/1
  Divide/1 -> Motordrehzahl/1

== system Library_ASK/Drehzahlrückführung az VA/Fall Zweiganggetriebe ==
  note: auf diese Weise wird die Goto/From - Rückführung aus dem EM -Block überflüssig
  Mittlere Raddrehzahl : Inport
  Enable : EnablePort
  Constant : Constant  Value=i_TRM_G1_VA
  Constant1 : Constant  Value=i_TRM_G2_VA
  Constant2 : Constant  Value=n_EM_max
  Divide : Product  Inputs=**
  Divide1 : Product  Inputs=**
  MATLAB Function : MATLAB Function  TreatAsAtomicUnit=on
  Motordrehzahl : Outport
  wires:
  Constant2/1 -> MATLAB Function/2(n_EM_max)
  Divide1/1 -> Motordrehzahl/1
  Constant1/1 -> MATLAB Function/4(i_TRM_G2)
  Divide/1 -> MATLAB Function/1(n_EM)  "Motordrehzahl wenn im ersten Gang"
  MATLAB Function/1(i_TRM) -> Divide1/2
  Mittlere Raddrehzahl/1 -> Divide1/1, Divide/1
  Constant/1 -> Divide/2, MATLAB Function/3(i_TRM_G1)

== system Library_ASK/Drehzahlrückführung rn HA/Fall Einganggetriebe ==
  Mittlere Raddrehzahl : Inport
  Enable : EnablePort
  Constant : Constant  Value=i_TRM_HA
  Divide : Product  Inputs=**
  Motordrehzahl : Outport
  wires:
  Constant/1 -> Divide/2
  Mittlere Raddrehzahl/1 -> Divide/1
  Divide/1 -> Motordrehzahl/1

== system Library_ASK/Drehzahlrückführung rn HA/Fall Zweiganggetriebe ==
  note: auf diese Weise wird die Goto/From - Rückführung aus dem EM -Block überflüssig
  note: Das ist jetzt tricky. Denn bei Kurvenfahrt kann es passieren, dass der eine Motor in den zweiten Gang schalten muss, der erste aber nicht.
  Raddrehzahl : Inport
  Enable : EnablePort
  Constant : Constant  Value=i_TRM_G1_HA
  Constant1 : Constant  Value=i_TRM_G2_HA
  Constant2 : Constant  Value=n_EM_max
  Demux : Demux  Outputs=2
  Divide : Product  Inputs=**
  Divide3 : Product  Inputs=**
  MATLAB Function : MATLAB Function  TreatAsAtomicUnit=on
  MATLAB Function1 : MATLAB Function  TreatAsAtomicUnit=on
  Mux : Mux  Inputs=2
  Motordrehzahl : Outport
  wires:
  Mux/1 -> Divide3/2
  Demux/2 -> MATLAB Function1/1(n_EM)  "Motor links"
  Demux/1 -> MATLAB Function/1(n_EM)  "Motor rechts"
  Constant2/1 -> MATLAB Function/2(n_EM_max), MATLAB Function1/2(n_EM_max)
  Constant1/1 -> MATLAB Function/4(i_TRM_G2), MATLAB Function1/4(i_TRM_G2)
  Divide/1 -> Demux/1  "Motordrehzahl wenn im ersten Gang"
  MATLAB Function/1(i_TRM) -> Mux/1
  Raddrehzahl/1 -> Divide3/1, Divide/1
  Constant/1 -> Divide/2, MATLAB Function/3(i_TRM_G1), MATLAB Function1/3(i_TRM_G1)
  MATLAB Function1/1(i_TRM) -> Mux/2
  Divide3/1 -> Motordrehzahl/1

== system Library_ASK/Drehzahlrückführung rn VA/Fall Einganggetriebe ==
  Raddrehzahl : Inport
  Enable : EnablePort
  Constant : Constant  Value=i_TRM_VA
  Divide : Product  Inputs=**
  Motordrehzahl : Outport
  wires:
  Divide/1 -> Motordrehzahl/1
  Raddrehzahl/1 -> Divide/1
  Constant/1 -> Divide/2

== system Library_ASK/Drehzahlrückführung rn VA/Fall Zweiganggetriebe ==
  note: Das ist jetzt tricky. Denn bei Kurvenfahrt kann es passieren, dass der eine Motor in den zweiten Gang schalten muss, der erste aber nicht.
  note: auf diese Weise wird die Goto/From - Rückführung aus dem EM -Block überflüssig
  Raddrehzahl : Inport
  Enable : EnablePort
  Constant : Constant  Value=i_TRM_G1_VA
  Constant1 : Constant  Value=i_TRM_G2_VA
  Constant2 : Constant  Value=n_EM_max
  Demux : Demux  Outputs=2
  Divide : Product  Inputs=**
  Divide2 : Product  Inputs=**
  MATLAB Function : MATLAB Function  TreatAsAtomicUnit=on
  MATLAB Function1 : MATLAB Function  TreatAsAtomicUnit=on
  Mux : Mux  Inputs=2
  Motordrehzahl : Outport
  wires:
  Constant/1 -> MATLAB Function1/3(i_TRM_G1), MATLAB Function/3(i_TRM_G1), Divide/2
  Raddrehzahl/1 -> Divide2/1, Divide/1
  MATLAB Function/1(i_TRM) -> Mux/1
  Divide/1 -> Demux/1  "Motordrehzahl wenn im ersten Gang"
  Constant1/1 -> MATLAB Function1/4(i_TRM_G2), MATLAB Function/4(i_TRM_G2)
  Constant2/1 -> MATLAB Function1/2(n_EM_max), MATLAB Function/2(n_EM_max)
  Demux/1 -> MATLAB Function/1(n_EM)  "Motor rechts"
  Demux/2 -> MATLAB Function1/1(n_EM)  "Motor links"
  Mux/1 -> Divide2/2
  MATLAB Function1/1(i_TRM) -> Mux/2
  Divide2/1 -> Motordrehzahl/1

== system Library_ASK/Elektrisches Überlagerungsgetriebe HA/Momentenkennlinie SEM ==
  Maximalmoment : Inport
  Drehzahl SteuerEM : Inport  Port=2
  Gain : Gain  Gain=-1
  M_Antr : Lookup_n-D  NumberOfTableDimensions=1  BreakpointsForDimension1=par_MDT.HA.trans.etv.Kennfelder.MaxMotorTrqCurve_w  Table=par_MDT.HA.trans.etv.Kennfelder.MaxMotorTrqCurve_M  ExtrapMethod=Clip  UseLastTableValue=on  InternalRulePriority=Speed  RndMeth=Simplest  InputSameDT=on
  M_Reku : Lookup_n-D  NumberOfTableDimensions=1  BreakpointsForDimension1=par_MDT.HA.trans.etv.Kennfelder.MaxGeneratorTrqCurve_w  Table=par_MDT.HA.trans.etv.Kennfelder.MaxGeneratorTrqCurve_M  ExtrapMethod=Clip  UseLastTableValue=on  InternalRulePriority=Speed  RndMeth=Simplest  InputSameDT=on
  Saturation Dynamic : simulink/Discontinuities/Saturation Dynamic  OutMin=[]  OutMax=[]  OutDataTypeStr=Inherit: Same as second input  OutDataType=fixdt(1, 16)  OutScaling=2^-10  DoSatur=off
  Maximalmoment bei Drehzahl : Outport
  wires:
  M_Antr/1 -> Saturation Dynamic/1
  Drehzahl SteuerEM/1 -> M_Antr/1, M_Reku/1
  Gain/1 -> Saturation Dynamic/3
  Maximalmoment/1 -> Saturation Dynamic/2
  Saturation Dynamic/1 -> Maximalmoment bei Drehzahl/1
  M_Reku/1 -> Gain/1

== system Library_ASK/Elektrisches Überlagerungsgetriebe HA/eUELG Steuermaschine ==
  Moment : Inport
  Drehzahl : Inport  Port=2
  Abs : Abs
  Abs1 : Abs
  Wirkungsgradkennfeld nach Pesce : Lookup_n-D  BreakpointsForDimension1=par_MDT.HA.trans.etv.Kennfelder.MotorEffMap3D_w  BreakpointsForDimension2=par_MDT.HA.trans.etv.Kennfelder.MotorEffMap3D_M  Table=par_MDT.HA.trans.etv.Kennfelder.MotorEffMap3D  ExtrapMethod=Clip  UseLastTableValue=on  InternalRulePriority=Speed  RndMeth=Simplest  InputSameDT=on
  Wirkungsgrad : Outport  InitialOutput=0
  wires:
  Moment/1 -> Abs/1
  Drehzahl/1 -> Abs1/1
  Wirkungsgradkennfeld nach Pesce/1 -> Wirkungsgrad/1
  Abs/1 -> Wirkungsgradkennfeld nach Pesce/2
  Abs1/1 -> Wirkungsgradkennfeld nach Pesce/1

== system Library_ASK/Elektrisches Überlagerungsgetriebe VA/Momentenkennlinie SEM ==
  Maximalmoment : Inport
  Drehzahl SteuerEM : Inport  Port=2
  Gain : Gain  Gain=-1
  M_Antr : Lookup_n-D  NumberOfTableDimensions=1  BreakpointsForDimension1=par_MDT.VA.trans.etv.Kennfelder.MaxMotorTrqCurve_w  Table=par_MDT.VA.trans.etv.Kennfelder.MaxMotorTrqCurve_M  ExtrapMethod=Clip  UseLastTableValue=on  InternalRulePriority=Speed  RndMeth=Simplest  InputSameDT=on
  M_Reku : Lookup_n-D  NumberOfTableDimensions=1  BreakpointsForDimension1=par_MDT.VA.trans.etv.Kennfelder.MaxGeneratorTrqCurve_w  Table=par_MDT.VA.trans.etv.Kennfelder.MaxGeneratorTrqCurve_M  ExtrapMethod=Clip  UseLastTableValue=on  InternalRulePriority=Speed  RndMeth=Simplest  InputSameDT=on
  Saturation Dynamic : simulink/Discontinuities/Saturation Dynamic  OutMin=[]  OutMax=[]  OutDataTypeStr=Inherit: Same as second input  OutDataType=fixdt(1, 16)  OutScaling=2^-10  DoSatur=off
  Maximalmoment bei Drehzahl : Outport
  wires:
  M_Reku/1 -> Gain/1
  Saturation Dynamic/1 -> Maximalmoment bei Drehzahl/1
  Maximalmoment/1 -> Saturation Dynamic/2
  Gain/1 -> Saturation Dynamic/3
  Drehzahl SteuerEM/1 -> M_Reku/1, M_Antr/1
  M_Antr/1 -> Saturation Dynamic/1

== system Library_ASK/Elektrisches Überlagerungsgetriebe VA/eUELG Steuermaschine ==
  Moment : Inport
  Drehzahl : Inport  Port=2
  Abs : Abs
  Abs1 : Abs
  Wirkungsgradkennfeld nach Pesce : Lookup_n-D  BreakpointsForDimension1=par_MDT.VA.trans.etv.Kennfelder.MotorEffMap3D_w  BreakpointsForDimension2=par_MDT.VA.trans.etv.Kennfelder.MotorEffMap3D_M  Table=par_MDT.VA.trans.etv.Kennfelder.MotorEffMap3D  ExtrapMethod=Clip  UseLastTableValue=on  InternalRulePriority=Speed  RndMeth=Simplest  InputSameDT=on
  Wirkungsgrad : Outport  InitialOutput=0
  wires:
  Abs1/1 -> Wirkungsgradkennfeld nach Pesce/1
  Abs/1 -> Wirkungsgradkennfeld nach Pesce/2
  Wirkungsgradkennfeld nach Pesce/1 -> Wirkungsgrad/1
  Drehzahl/1 -> Abs1/1
  Moment/1 -> Abs/1

== system Library_ASK/Kelly/x-Achsen-Parameter ==
  note: Umfangskraft Planententeilkreis
  Drehzahl Planet : Inport
  Teilkreis Planet : Inport  Port=2
  Stegmoment : Inport  Port=3
  Durchmesser Steg : Inport  Port=4
  Constant1 : Constant  Value=2
  Divide1 : Product  Inputs=*/
  Eingriffswinkel : Constant  Value=alpha
  Gain2 : Gain  Gain=0.5
  "N/mm -> lb/in" : Gain  Gain=5.71
  "Nm -> Nmm" : Gain  Gain=1000
  Product : Product  Inputs=3
  Product3 : Product
  Summengeschwindigkeit : Product  Inputs=3
  Trigonometric Function1 : Trigonometry
  Zahnbreite : Constant  Value=b_zahn
  "m/s -> in/s" : Gain  Gain=39.37
  max. 50m/s : Saturate  UpperLimit=50  LowerLimit=0
  "mm -> m" : Gain  Gain=0.001
  mu0 : Constant  Value=0.1
  normal load : Product  Inputs=*/
  mu0*vs/W : Outport
  wires:
  Zahnbreite/1 -> normal load/2
  Product3/1 -> max. 50m/s/1
  Divide1/1 -> Gain2/1
  Durchmesser Steg/1 -> Divide1/2
  Eingriffswinkel/1 -> Trigonometric Function1/1
  Constant1/1 -> Summengeschwindigkeit/2
  "Nm -> Nmm"/1 -> Divide1/1
  Stegmoment/1 -> "Nm -> Nmm"/1
  "mm -> m"/1 -> Product3/1
  max. 50m/s/1 -> Summengeschwindigkeit/1
  Trigonometric Function1/1 -> Summengeschwindigkeit/3
  mu0/1 -> Product/3
  Summengeschwindigkeit/1 -> "m/s -> in/s"/1
  Drehzahl Planet/1 -> Product3/2
  Teilkreis Planet/1 -> "mm -> m"/1
  normal load/1 -> "N/mm -> lb/in"/1
  Gain2/1 -> normal load/1
  Product/1 -> mu0*vs/W/1
  "N/mm -> lb/in"/1 -> Product/2
  "m/s -> in/s"/1 -> Product/1

== system Library_ASK/Leistungselektronik/Powerfactorberechnung ==
  Drehmoment : Inport
  Drehzahl : Inport  Port=2
  2-D Lookup Table : Lookup_n-D  BreakpointsForDimension1=Torque  BreakpointsForDimension2=Speed  Table=Powerfactor_Map  ExtrapMethod=Clip  UseLastTableValue=on  InternalRulePriority=Speed  RndMeth=Simplest  InputSameDT=on
  Powerfactor : Outport
  wires:
  Drehzahl/1 -> 2-D Lookup Table/2
  2-D Lookup Table/1 -> Powerfactor/1
  Drehmoment/1 -> 2-D Lookup Table/1

== system Library_ASK/Leistungselektronik/Stromberechnung ==
  Leistung : Inport
  Spannung : Inport  Port=2
  Powerfactor : Inport  Port=3
  Constant1 : Constant  Value=3
  Divide : Product  Inputs=*///
  Strom : Outport
  wires:
  Powerfactor/1 -> Divide/4
  Constant1/1 -> Divide/2
  Leistung/1 -> Divide/1
  Spannung/1 -> Divide/3
  Divide/1 -> Strom/1

== system Library_ASK/Leistungselektronik/Wirkungsgradberechnung ==
  Strom : Inport
  Spannung : Inport  Port=2
  Powerfactor : Inport  Port=3
  n-D Lookup Table : Lookup_n-D  NumberOfTableDimensions=3  BreakpointsForDimension1=Current  BreakpointsForDimension2=Voltage  BreakpointsForDimension3=Powerfactor  Table=Efficiency_Map  ExtrapMethod=Clip  UseLastTableValue=on  InternalRulePriority=Speed  RndMeth=Simplest  InputSameDT=on
  Wirkungsgrad_LE : Outport
  wires:
  n-D Lookup Table/1 -> Wirkungsgrad_LE/1
  Strom/1 -> n-D Lookup Table/1
  Powerfactor/1 -> n-D Lookup Table/3
  Spannung/1 -> n-D Lookup Table/2

== system Library_ASK/Limited Slip Differential/Kupplung ==
  M_TV_Wunsch : Inport
  okay : Inport  Port=2
  Restrict M_TV : Inport  Port=3
  Constant1 : Constant  Value=0
  Divide1 : Product  Inputs=*/**
  Fx_max : Constant  Value=Fx_LSD_max
  Gain : Gain  Gain=-1
  Gain1 : Gain  Gain=0.5
  M-Cl-max : Constant  Value=M_Cl_LSD_max
  PT1_LSD : DiscreteTransferFcn  Numerator=[0 4.9988e-04]  Denominator=[1 -0.9995]
  Product : Product  Inputs=4
  Reibflächen : Constant  Value=nreib_LSD
  Saturation Dynamic : simulink/Discontinuities/Saturation Dynamic  OutMin=[]  OutMax=[]  OutDataTypeStr=Inherit: Same as second input  OutDataType=fixdt(1, 16)  OutScaling=2^-10  DoSatur=off
  Saturation Dynamic1 : simulink/Discontinuities/Saturation Dynamic  OutMin=[]  OutMax=[]  OutDataTypeStr=Inherit: Same as second input  OutDataType=fixdt(1, 16)  OutScaling=2^-10  DoSatur=off
  Zero-Order Hold2 : ZeroOrderHold  SampleTime=stepsize
  mu_cl : Constant  Value=mu_cl_LSD
  rm : Constant  Value=rm_LSD
  M_Kupplung : Outport
  M_Kuppl_Wunsch : Outport  Port=2
  wires:
  M-Cl-max/1 -> Divide1/2
  Fx_max/1 -> Saturation Dynamic/1, Divide1/3
  Constant1/1 -> Saturation Dynamic/3
  Divide1/1 -> Saturation Dynamic/2  "Fx_Wunsch"
  Zero-Order Hold2/1 -> PT1_LSD/1
  mu_cl/1 -> Product/3
  rm/1 -> Product/2
  Product/1 -> M_Kupplung/1
  Reibflächen/1 -> Product/4
  okay/1 -> Divide1/4
  PT1_LSD/1 -> Product/1
  Saturation Dynamic/1 -> Zero-Order Hold2/1
  M_TV_Wunsch/1 -> Gain1/1
  Saturation Dynamic1/1 -> Divide1/1
  Restrict M_TV/1 -> Saturation Dynamic1/1, Gain/1
  Gain/1 -> Saturation Dynamic1/3
  Gain1/1 -> M_Kuppl_Wunsch/1, Saturation Dynamic1/2  "M_Kuppl_Wunsch"

== system Library_ASK/Limited Slip Differential/Reifenmodellvoraussage ==
  nri : Inport
  nli : Inport  Port=2
  Reifenaufstandskraft : Inport  Port=3
  r_dyn : Inport  Port=4
  Fahrzeuggeschwindigkeit : Inport  Port=5
  Abs2 : Abs
  Add2 : Sum  Inputs=-+
  Divide1 : Product  Inputs=****/*
  Gain : Gain  Gain=0.5
  MinMax : MinMax
  Reifenlängssteifigkeit bei Schlupf = 0 : Constant  Value=20
  M_Kupplung_grenz : Outport
  wires:
  Add2/1 -> Abs2/1
  Abs2/1 -> Gain/1
  Gain/1 -> Divide1/1
  Reifenlängssteifigkeit bei Schlupf = 0/1 -> Divide1/6
  r_dyn/1 -> Divide1/4, Divide1/3
  Fahrzeuggeschwindigkeit/1 -> Divide1/5
  Reifenaufstandskraft/1 -> Divide1/2
  Divide1/1 -> MinMax/1
  MinMax/1 -> M_Kupplung_grenz/1
  nri/1 -> Add2/1
  nli/1 -> Add2/2

== system Library_ASK/Limited Slip Differential -- alt/MATLAB Function ==
  M_D : Inport
  M_Sperr : Inport  Port=2
  " Demux " : Demux  Outputs=1
  " SFunction " : S-Function  Tag=Stateflow S-Function Library_Antriebsstrangkomponenten 2  FunctionName=sf_sfun  PortCounts=[2 3]  SFunctionDeploymentMode=off  EnableBusSupport=off
  " Terminator " : Terminator
  M_S : Outport
  M_Right_Wheel : Outport  Port=2
  wires:
  " SFunction "/1 -> " Demux "/1
  " Demux "/1 -> " Terminator "/1
  " SFunction "/3 -> M_Right_Wheel/1  "M_Right_Wheel"
  " SFunction "/2 -> M_S/1  "M_S"
  M_Sperr/1 -> " SFunction "/2
  M_D/1 -> " SFunction "/1

== system Library_ASK/Mehrstufiges Getriebe HA/Subsystem ==
  WKG : Inport
  Inputleistung : Inport  Port=2
  Abs : Abs
  Add : Sum  Inputs=+-
  Constant : Constant
  Discrete-Time Integrator : DiscreteIntegrator  gainval=1  SampleTime=-1  ICPrevOutput=DiscIntNeverNeededParam  ICPrevScaledInput=DiscIntNeverNeededParam
  Product5 : Product
  "W -> kW" : Gain  Gain=0.001
  "Ws -> kWh" : Gain  Gain=1/3600000
  Energieverlust [kWh] : Outport
  Verlustleistung [kW] : Outport  Port=2
  wires:
  Constant/1 -> Add/1
  Inputleistung/1 -> Product5/2
  Add/1 -> Product5/1
  Discrete-Time Integrator/1 -> "Ws -> kWh"/1
  "Ws -> kWh"/1 -> Energieverlust [kWh]/1
  Abs/1 -> "W -> kW"/1, Discrete-Time Integrator/1
  Product5/1 -> Abs/1
  "W -> kW"/1 -> Verlustleistung [kW]/1
  WKG/1 -> Add/2

== system Library_ASK/Mehrstufiges Getriebe HA/WKG ==
  note: maximaler Wert im Table im init_MVS auf eta_aa festgelegt
  Stufenübersetzung : Inport
  Stufenanzahl : Inport  Port=2
  Eingangsdrehzahl : Inport  Port=3
  Last : Inport  Port=4
  Stufenübersetzung2 : Inport  Port=5
  1-D Lookup Table Stufe 1 : Lookup_n-D  NumberOfTableDimensions=1  BreakpointsForDimension1=breakpointset  Table=wkg_GTR  InternalRulePriority=Speed  RndMeth=Simplest  InputSameDT=on
  Math Function : Math  Operator=pow  SaturateOnIntegerOverflow=on
  Terminator{,1..3} (4 alike) : Terminator
  WKG : Outport
  wires:
  Stufenübersetzung2/1 -> Terminator3/1
  Eingangsdrehzahl/1 -> Terminator/1
  Math Function/1 -> WKG/1
  1-D Lookup Table Stufe 1/1 -> Math Function/1
  Stufenanzahl/1 -> Terminator2/1, Math Function/2
  Stufenübersetzung/1 -> Terminator1/1
  Last/1 -> 1-D Lookup Table Stufe 1/1

== system Library_ASK/Mehrstufiges Getriebe VA/Subsystem ==
  WKG : Inport
  Inputleistung : Inport  Port=2
  Abs : Abs
  Add : Sum  Inputs=+-
  Constant : Constant
  Discrete-Time Integrator : DiscreteIntegrator  gainval=1  SampleTime=-1  ICPrevOutput=DiscIntNeverNeededParam  ICPrevScaledInput=DiscIntNeverNeededParam
  Product5 : Product
  "W -> kW" : Gain  Gain=0.001
  "Ws -> kWh" : Gain  Gain=1/3600000
  Energieverlust [kWh] : Outport
  Verlustleistung [kW] : Outport  Port=2
  wires:
  WKG/1 -> Add/2
  "W -> kW"/1 -> Verlustleistung [kW]/1
  Product5/1 -> Abs/1
  Abs/1 -> Discrete-Time Integrator/1, "W -> kW"/1
  "Ws -> kWh"/1 -> Energieverlust [kWh]/1
  Discrete-Time Integrator/1 -> "Ws -> kWh"/1
  Add/1 -> Product5/1
  Inputleistung/1 -> Product5/2
  Constant/1 -> Add/1

== system Library_ASK/Mehrstufiges Getriebe VA/WKG ==
  note: Geometriewerte kommen dann aus par_VEH
  note: diese Getriebe übersetzen immer ins Langsame, daher ist die Eingangsdrehzahl immer die Ritzeldrehzahl
  note: maximaler Wert im Table im init_MVS auf eta_aa festgelegt
  Stufenübersetzung 1 : Inport
  Stufenanzahl : Inport  Port=2
  Eingangsdrehzahl : Inport  Port=3
  Last : Inport  Port=4
  Stufenübersetzung 2 : Inport  Port=5
  Eingangsmoment : Inport  Port=6
  1-D Lookup Table Stufe 1 : Lookup_n-D  NumberOfTableDimensions=1  BreakpointsForDimension1=breakpointset  Table=wkg_GTR  InternalRulePriority=Speed  RndMeth=Simplest  InputSameDT=on
  Constant : Constant  Value=25
  Constant{1..2,4..5} (4 alike) : Constant  Value=50
  Constant3 : Constant  Value=10
  Divide : Product  Inputs=*/
  Math Function : Math  Operator=pow  SaturateOnIntegerOverflow=on
  NWH Stufengetriebe : $bdroot/NWH Stufengetriebe  SystemSampleTime=-1
  NWH Stufengetriebe1 : $bdroot/NWH Stufengetriebe  SystemSampleTime=-1
  Product : Product  Inputs=***
  Product1 : Product
  Scope : Scope
  Scope1 : Scope
  Übersetzungsabhängiger Maximalwirkugsgrad : Subsystem
  WKG Pesce : Outport
  WKG NWH : Outport  Port=2
  wires:
  Stufenübersetzung 1/1 -> Divide/2, NWH Stufengetriebe/1, Product/2
  Stufenanzahl/1 -> Math Function/2
  1-D Lookup Table Stufe 1/1 -> Math Function/1
  Math Function/1 -> WKG Pesce/1
  Eingangsdrehzahl/1 -> Divide/1, NWH Stufengetriebe/2
  Stufenübersetzung 2/1 -> NWH Stufengetriebe1/1
  Eingangsmoment/1 -> Product/1, NWH Stufengetriebe/3
  Constant/1 -> NWH Stufengetriebe/4
  Constant1/1 -> NWH Stufengetriebe/5
  Constant2/1 -> NWH Stufengetriebe1/5
  Constant3/1 -> NWH Stufengetriebe1/4
  NWH Stufengetriebe/1 -> Product1/1, Product/3
  Product/1 -> NWH Stufengetriebe1/3
  Divide/1 -> NWH Stufengetriebe1/2
  NWH Stufengetriebe/2 -> Scope/1
  NWH Stufengetriebe1/2 -> Scope1/1
  NWH Stufengetriebe1/1 -> Product1/2
  Product1/1 -> WKG NWH/1
  Constant4/1 -> NWH Stufengetriebe/6
  Constant5/1 -> NWH Stufengetriebe1/6
  Last/1 -> 1-D Lookup Table Stufe 1/1
